simulink model "cw5_model_BORKOWSKI_17"  (R2024a)
settings: Solver=VariableStepAuto  StartTime=0.0  StopTime=10.0  MaxStep=0.01  MinStep=0.001  RelTol=1e-6
values from neighbouring files (symbols this model uses):
  A = [0 1;-a0 -a1]    [cw5_dane_BORKOWSKI.m]
  a0 = h/m    (= 6.25)    [cw5_dane_BORKOWSKI.m]
  a1 = a/m    (= 0.625)    [cw5_dane_BORKOWSKI.m]
  B = [0;b0]    [cw5_dane_BORKOWSKI.m]
  b0 = 1/m    (= 15.625)    [cw5_dane_BORKOWSKI.m]
  C = [1 0]    [cw5_dane_BORKOWSKI.m]
  D = [0]    [cw5_dane_BORKOWSKI.m]
settings Model: Creator=Student  LastModifiedBy=Kamil
settings SolverCC: AlgebraicLoopSolver=TrustRegion
settings DataIOCC: SaveFormat=Array  ReturnWorkspaceOutputs=off
settings DebuggingCC: ArithmeticOperatorsInVariantConditions=warning
settings SFSimCC: CustomCodeUndefinedFunction=UseInterfaceOnly
settings RTWCC: GPUComputeCapability=3.5
settings CodeAppCC: StateflowObjectComments=on

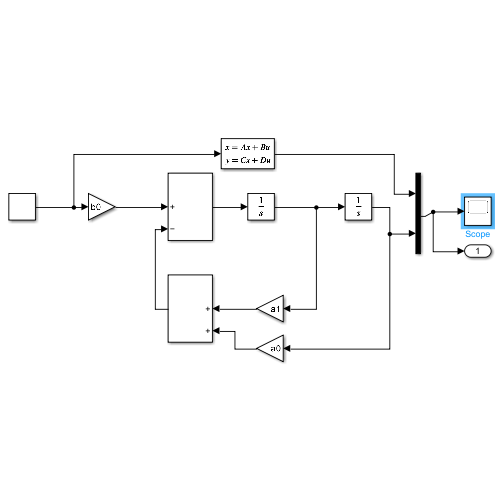
[thumbnail: Simulink's stored preview of the top-level diagram]
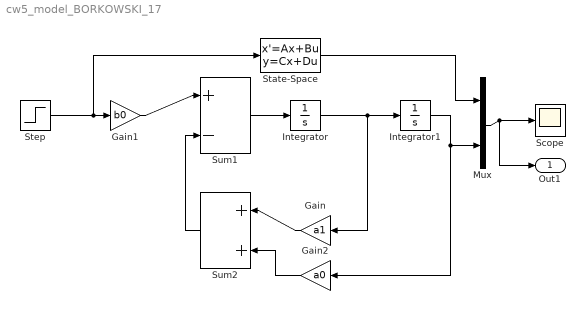
== system cw5_model_BORKOWSKI_17 ==
  Gain : Gain  Gain=a1
  Gain1 : Gain  Gain=b0
  Gain2 : Gain  Gain=a0
  Integrator : Integrator
  Integrator1 : Integrator
  Mux : Mux  Inputs=2
  Scope : Scope
  State-Space : StateSpace  A=A  B=B  C=C  D=D  InitialCondition=0
  Step : Step  Time=0  Before=1  SampleTime=0
  Sum1 : Sum  Inputs=|+-
  Sum2 : Sum  Inputs=|++
  Out1 : Outport
  wires:
  Mux/1 -> Out1/1, Scope/1
  Integrator1/1 -> Gain2/1, Mux/2
  Integrator/1 -> Gain/1, Integrator1/1
  Sum1/1 -> Integrator/1
  Gain1/1 -> Sum1/1
  Step/1 -> State-Space/1, Gain1/1
  Sum2/1 -> Sum1/2
  Gain/1 -> Sum2/1
  Gain2/1 -> Sum2/2
  State-Space/1 -> Mux/1
